simulink model "s1213_91"  (R2018a)
settings: Solver=VariableStepAuto  StartTime=0.0  StopTime=10.0  RelTol=1e-3
settings Model: Creator=Administrator  LastModifiedBy=Administrator
settings DataIOCC: ReturnWorkspaceOutputs=on
settings SFSimCC: SimUseLocalCustomCode=on
settings RTWCC: RTWUseLocalCustomCode=on

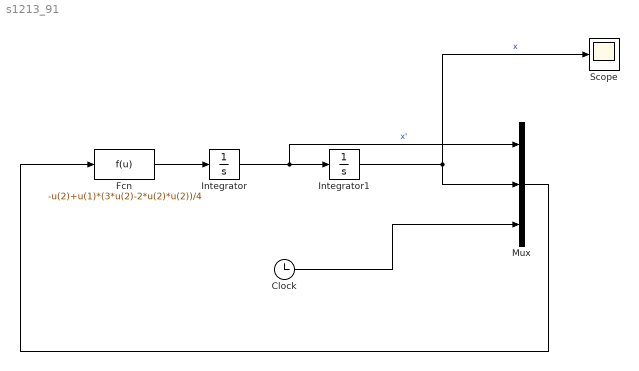
== system s1213_91 ==
  Clock : Clock
  Fcn : Fcn  Expr=-u(2)+u(1)*(3*u(2)-2*u(2)*u(2))/4
  Integrator : Integrator  InitialCondition=1
  Integrator1 : Integrator  InitialCondition=2
  Mux : Mux  Inputs=3
  Scope : Scope
  wires:
  Integrator/1 -> Mux/1, Integrator1/1  "x'"
  Integrator1/1 -> Mux/2, Scope/1  "x"
  Mux/1 -> Fcn/1
  Clock/1 -> Mux/3
  Fcn/1 -> Integrator/1
